simulink model "Vorlage_Prozessgut_Jaeho"  (R2022a)
settings: Solver=ode3  StartTime=0.0  StopTime=50  FixedStep=0.01  RelTol=1e-3  EnableMultiTasking=on
undefined symbols (not defined in the file): MaxFlaschen
libraries: simulink x19
settings Model: Creator=merz  LastModifiedBy=mwjae
settings SolverCC: ZeroCrossAlgorithm=Non-adaptive  AlgebraicLoopSolver=TrustRegion
settings DataIOCC: LimitDataPoints=on  SaveFormat=Array  SignalLoggingSaveFormat=ModelDataLogs  ReturnWorkspaceOutputs=off  SignalLoggingName=sigsOut
settings OptimizationCC: ExpressionDepthLimit=2147483647  InitFltsAndDblsToZero=on  LifeSpan=inf
settings DebuggingCC: SaveWithParameterizedLinksMsg=none  UnderspecifiedInitializationDetection=Classic  MergeDetectMultiDrivingBlocksExec=none  SignalResolutionControl=TryResolveAllWithWarning  MultiTaskDSMMsg=warning  MultiTaskCondExecSysMsg=none  FcnCallInpInsideContextMsg=warning  UnconnectedInputMsg=warning  UnconnectedOutputMsg=warning  UnconnectedLineMsg=warning  StateNameClashWarn=warning  SFUnexpectedBacktrackingDiag=warning  SFNoUnconditionalDefaultTransitionDiag=warning  SFExecutionAtInitializationDiag=none  SFMachineParentedDataDiag=warning  ArithmeticOperatorsInVariantConditions=warning
settings HardwareCC: ProdBitPerPointer=32  ProdBitPerSizeT=32  ProdBitPerPtrDiffT=32  ProdLargestAtomicFloat=None  ProdIntDivRoundTo=Undefined  ProdEndianess=Unspecified  ProdWordSize=32  ProdHWDeviceType=32-bit Generic  TargetUnknown=on
settings ModelReferenceCC: PropagateSignalLabelsOutOfModel=off
settings RTWCC: DLArmComputeVersion=19.05
settings CodeAppCC: StateflowObjectComments=on
settings GRTTargetCC: TargetFcnLib=ansi_tfl_tmw.mat  TargetLangStandard=C89/C90 (ANSI)  ModelReferenceCompliant=off  CombineOutputUpdateFcns=off  MatFileLogging=off  GRTInterface=on
settings ConfigComp: CovMetricSettings=dw  CovSaveCumulativeToWorkspaceVar=on  CovSaveSingleToWorkspaceVar=on

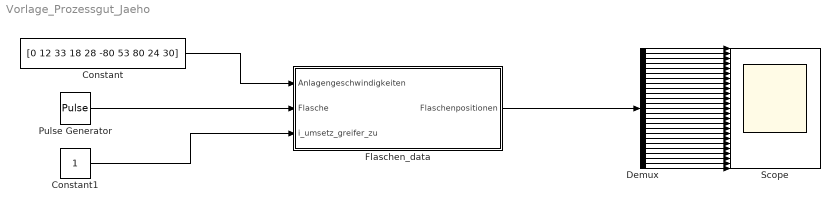
== system Vorlage_Prozessgut_Jaeho ==
  Constant : Constant  Value=[0 12 33 18 28 -80 53 80 24 30]
  Constant1 : Constant
  Demux : Demux  Outputs=25
  Flaschen_data : Subsystem
  Pulse Generator : DiscretePulseGenerator  PulseType=Time based  PulseWidth=10
  Scope : Scope  NumInputPorts=25
  wires:
  Pulse Generator/1 -> Flaschen_data/2(Flasche)
  Constant1/1 -> Flaschen_data/3(i_umsetz_greifer_zu)
  Constant/1 -> Flaschen_data/1(Anlagengeschwindigkeiten)
  Demux/2 -> Scope/2
  Demux/22 -> Scope/22
  Demux/16 -> Scope/16
  Demux/20 -> Scope/20
  Demux/5 -> Scope/5
  Demux/7 -> Scope/7
  Demux/19 -> Scope/19
  Demux/10 -> Scope/10
  Demux/9 -> Scope/9
  Demux/17 -> Scope/17
  Demux/15 -> Scope/15
  Demux/11 -> Scope/11
  Demux/8 -> Scope/8
  Demux/6 -> Scope/6
  Demux/3 -> Scope/3
  Demux/13 -> Scope/13
  Demux/25 -> Scope/25
  Demux/14 -> Scope/14
  Demux/1 -> Scope/1
  Demux/24 -> Scope/24
  Demux/4 -> Scope/4
  Demux/18 -> Scope/18
  Flaschen_data/1(Flaschenpositionen) -> Demux/1
  Demux/23 -> Scope/23
  Demux/12 -> Scope/12
  Demux/21 -> Scope/21

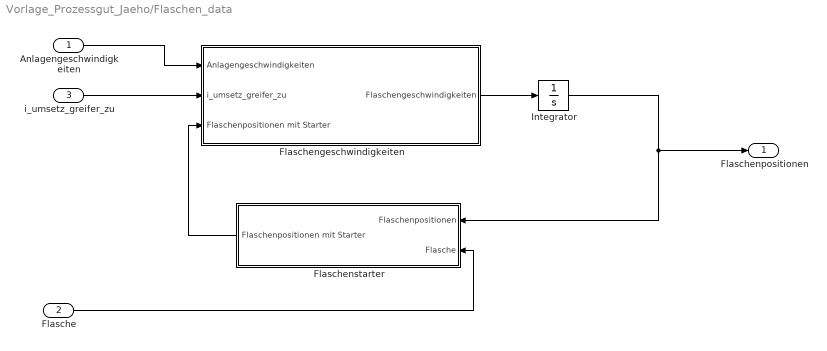
== system Vorlage_Prozessgut_Jaeho/Flaschen_data ==
  Anlagengeschwindigkeiten : Inport
  Flasche : Inport  Port=2
  i_umsetz_greifer_zu : Inport  Port=3
  Flaschengeschwindigkeiten : Subsystem
  Flaschenstarter : Subsystem
  Integrator : Integrator
  Flaschenpositionen : Outport
  wires:
  Anlagengeschwindigkeiten/1 -> Flaschengeschwindigkeiten/1(Anlagengeschwindigkeiten)
  i_umsetz_greifer_zu/1 -> Flaschengeschwindigkeiten/2(i_umsetz_greifer_zu)
  Flaschenstarter/1(Flaschenpositionen mit Starter) -> Flaschengeschwindigkeiten/3(Flaschenpositionen mit Starter)
  Flasche/1 -> Flaschenstarter/2(Flasche)
  Flaschengeschwindigkeiten/1(Flaschengeschwindigkeiten) -> Integrator/1
  Integrator/1 -> Flaschenstarter/1(Flaschenpositionen), Flaschenpositionen/1

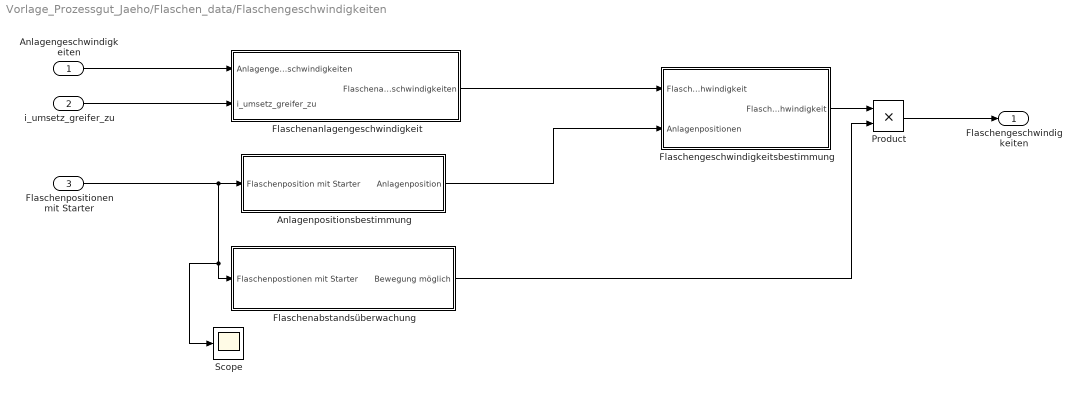
== system Vorlage_Prozessgut_Jaeho/Flaschen_data/Flaschengeschwindigkeiten ==
  Anlagengeschwindigkeiten : Inport
  i_umsetz_greifer_zu : Inport  Port=2
  Flaschenpositionen mit Starter : Inport  Port=3
  Anlagenpositionsbestimmung : Subsystem
  Flaschenabstandsüberwachung : Subsystem
  Flaschenanlagengeschwindigkeit : Subsystem
  "Flaschengeschwindigkeitsbestimmung " : Subsystem  TreatAsAtomicUnit=on
  Product : Product
  Scope : Scope
  Flaschengeschwindigkeiten : Outport
  wires:
  Anlagengeschwindigkeiten/1 -> Flaschenanlagengeschwindigkeit/1(Anlagengeschwindigkeiten)
  i_umsetz_greifer_zu/1 -> Flaschenanlagengeschwindigkeit/2(i_umsetz_greifer_zu)
  Flaschenanlagengeschwindigkeit/1(Flaschenanlagengeschwindigkeiten) -> "Flaschengeschwindigkeitsbestimmung "/1(Flaschenanlagengeschwindigkeit)
  Anlagenpositionsbestimmung/1(Anlagenposition) -> "Flaschengeschwindigkeitsbestimmung "/2(Anlagenpositionen)
  Flaschenpositionen mit Starter/1 -> Scope/1, Flaschenabstandsüberwachung/1(Flaschenpostionen mit Starter), Anlagenpositionsbestimmung/1(Flaschenposition mit Starter)
  "Flaschengeschwindigkeitsbestimmung "/1(Flaschengeschwindigkeit) -> Product/1
  Flaschenabstandsüberwachung/1(Bewegung möglich) -> Product/2
  Product/1 -> Flaschengeschwindigkeiten/1

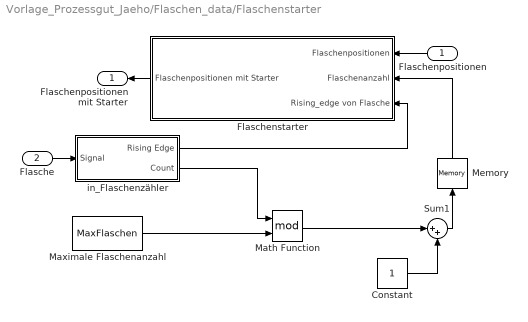
== system Vorlage_Prozessgut_Jaeho/Flaschen_data/Flaschenstarter ==
  Flaschenpositionen : Inport
  Flasche : Inport  Port=2
  Constant : Constant  OutDataTypeStr=uint16
  Flaschenstarter : Subsystem
  Math Function : Math  Operator=mod  SignedPower=on
  Maximale Flaschenanzahl : Constant  Value=MaxFlaschen  OutDataTypeStr=uint16
  Memory : Memory  InitialCondition=1
  Sum1 : Sum  Inputs=|++  SaturateOnIntegerOverflow=on
  in_Flaschenzähler : Subsystem
  Flaschenpositionen mit Starter : Outport
  wires:
  in_Flaschenzähler/2(Count) -> Math Function/1
  Maximale Flaschenanzahl/1 -> Math Function/2
  Math Function/1 -> Sum1/1
  in_Flaschenzähler/1(Rising Edge) -> Flaschenstarter/3(Rising_edge von Flasche)
  Sum1/1 -> Memory/1
  Constant/1 -> Sum1/2
  Memory/1 -> Flaschenstarter/2(Flaschenanzahl)
  Flaschenpositionen/1 -> Flaschenstarter/1(Flaschenpositionen)
  Flaschenstarter/1(Flaschenpositionen mit Starter) -> Flaschenpositionen mit Starter/1
  Flasche/1 -> in_Flaschenzähler/1(Signal)

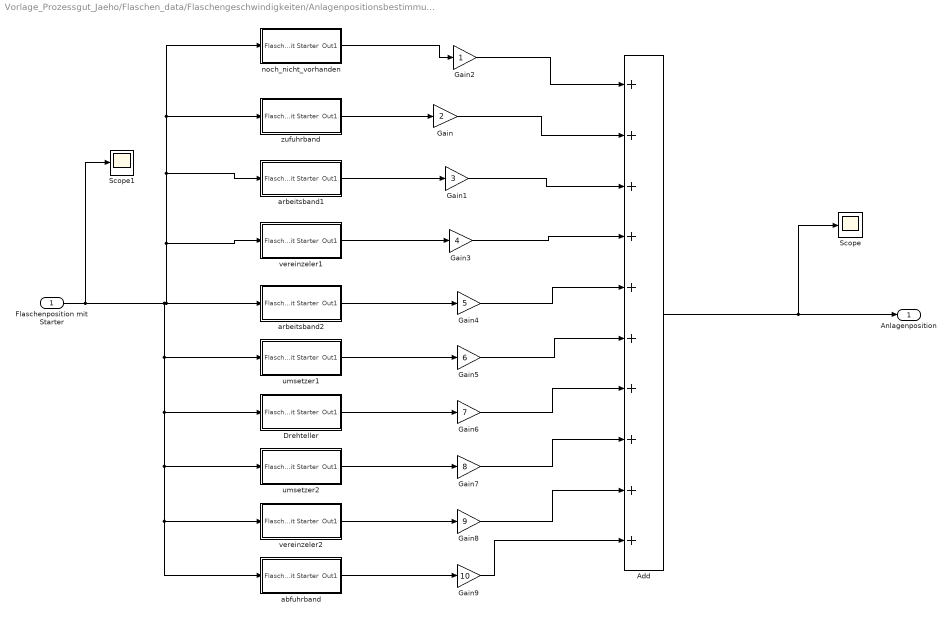
== system Vorlage_Prozessgut_Jaeho/Flaschen_data/Flaschengeschwindigkeiten/Anlagenpositionsbestimmung ==
  Flaschenposition mit Starter : Inport
  Add : Sum  Inputs=++++++++++
  Drehteller : Subsystem
  Gain : Gain  Gain=2
  Gain1 : Gain  Gain=3
  Gain2 : Gain
  Gain3 : Gain  Gain=4
  Gain4 : Gain  Gain=5
  Gain5 : Gain  Gain=6
  Gain6 : Gain  Gain=7
  Gain7 : Gain  Gain=8
  Gain8 : Gain  Gain=9
  Gain9 : Gain  Gain=10
  Scope : Scope
  Scope1 : Scope
  abfuhrband : Subsystem
  arbeitsband1 : Subsystem
  arbeitsband2 : Subsystem
  noch_nicht_vorhanden : Subsystem
  umsetzer1 : Subsystem
  umsetzer2 : Subsystem
  vereinzeler1 : Subsystem
  vereinzeler2 : Subsystem
  zufuhrband : Subsystem
  Anlagenposition : Outport
  wires:
  Flaschenposition mit Starter/1 -> Scope1/1, abfuhrband/1(Flaschenposition mit Starter), vereinzeler2/1(Flaschenposition mit Starter), umsetzer2/1(Flaschenposition mit Starter), Drehteller/1(Flaschenposition mit Starter), umsetzer1/1(Flaschenposition mit Starter), vereinzeler1/1(Flaschenposition mit Starter), arbeitsband1/1(Flaschenposition mit Starter), zufuhrband/1(Flaschenposition mit Starter), noch_nicht_vorhanden/1(Flaschenposition mit Starter), arbeitsband2/1(Flaschenposition mit Starter)
  Add/1 -> Scope/1, Anlagenposition/1
  Gain/1 -> Add/2
  Gain1/1 -> Add/3
  Gain2/1 -> Add/1
  Gain3/1 -> Add/4
  Gain4/1 -> Add/5
  Gain5/1 -> Add/6
  Gain6/1 -> Add/7
  Gain7/1 -> Add/8
  Gain8/1 -> Add/9
  Gain9/1 -> Add/10
  noch_nicht_vorhanden/1(Out1) -> Gain2/1
  zufuhrband/1(Out1) -> Gain/1
  arbeitsband1/1(Out1) -> Gain1/1
  vereinzeler1/1(Out1) -> Gain3/1
  arbeitsband2/1(Out1) -> Gain4/1
  umsetzer1/1(Out1) -> Gain5/1
  Drehteller/1(Out1) -> Gain6/1
  umsetzer2/1(Out1) -> Gain7/1
  vereinzeler2/1(Out1) -> Gain8/1
  abfuhrband/1(Out1) -> Gain9/1

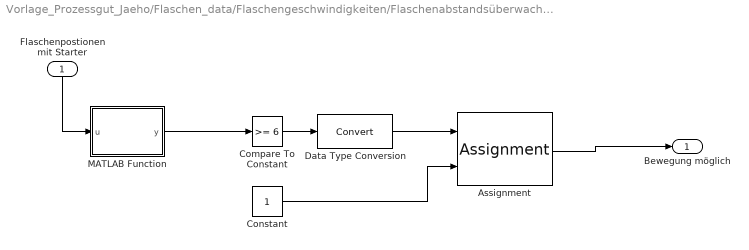
== system Vorlage_Prozessgut_Jaeho/Flaschen_data/Flaschengeschwindigkeiten/Flaschenabstandsüberwachung ==
  Flaschenpostionen mit Starter : Inport
  Assignment : Assignment  DiagnosticForDimensions=Warning  IndexOptions=Index vector (dialog)  Indices=1  OutputSizes=1
  Compare To Constant : simulink/Logic and Bit Operations/Compare To Constant  relop=>=  const=6  OutDataTypeStr=boolean
  Constant : Constant
  Data Type Conversion : DataTypeConversion  SaturateOnIntegerOverflow=off  RndMeth=Floor
  MATLAB Function : MATLAB Function  TreatAsAtomicUnit=on
  Bewegung möglich : Outport
  wires:
  Flaschenpostionen mit Starter/1 -> MATLAB Function/1(u)
  MATLAB Function/1(y) -> Compare To Constant/1
  Compare To Constant/1 -> Data Type Conversion/1
  Constant/1 -> Assignment/2
  Assignment/1 -> Bewegung möglich/1
  Data Type Conversion/1 -> Assignment/1

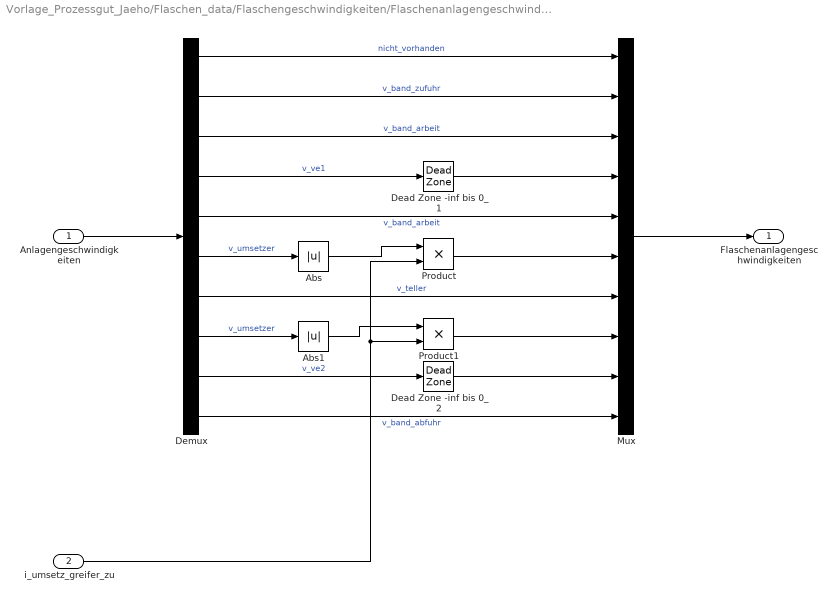
== system Vorlage_Prozessgut_Jaeho/Flaschen_data/Flaschengeschwindigkeiten/Flaschenanlagengeschwindigkeit ==
  Anlagengeschwindigkeiten : Inport
  i_umsetz_greifer_zu : Inport  Port=2
  Abs : Abs  SaturateOnIntegerOverflow=off
  Abs1 : Abs  SaturateOnIntegerOverflow=off
  Dead Zone -inf bis 0_1 : DeadZone  LowerValue=-inf  UpperValue=0
  Dead Zone -inf bis 0_2 : DeadZone  LowerValue=-inf  UpperValue=0
  Demux : Demux  Outputs=10
  Mux : Mux  Inputs=10
  Product : Product
  Product1 : Product
  Flaschenanlagengeschwindigkeiten : Outport
  wires:
  Anlagengeschwindigkeiten/1 -> Demux/1
  Demux/1 -> Mux/1  "nicht_vorhanden"
  Demux/2 -> Mux/2  "v_band_zufuhr"
  Demux/3 -> Mux/3  "v_band_arbeit"
  Demux/4 -> Dead Zone -inf bis 0_1/1  "v_ve1"
  Demux/5 -> Mux/5  "v_band_arbeit"
  Demux/6 -> Abs/1  "v_umsetzer"
  Demux/7 -> Mux/7  "v_teller"
  Demux/8 -> Abs1/1  "v_umsetzer"
  Demux/10 -> Mux/10  "v_band_abfuhr"
  Dead Zone -inf bis 0_1/1 -> Mux/4
  Dead Zone -inf bis 0_2/1 -> Mux/9
  Demux/9 -> Dead Zone -inf bis 0_2/1  "v_ve2"
  Abs/1 -> Product/1
  i_umsetz_greifer_zu/1 -> Product1/2, Product/2
  Abs1/1 -> Product1/1
  Product/1 -> Mux/6
  Product1/1 -> Mux/8
  Mux/1 -> Flaschenanlagengeschwindigkeiten/1

== system Vorlage_Prozessgut_Jaeho/Flaschen_data/Flaschengeschwindigkeiten/Flaschengeschwindigkeitsbestimmung  ==
  Flaschenanlagengeschwindigkeit : Inport
  Anlagenpositionen : Inport  Port=2
  Selector : Selector  InputPortWidth=10  IndexOptions=Index vector (port)  Indices=[1 3]  OutputSizes=1
  Flaschengeschwindigkeit : Outport
  wires:
  Flaschenanlagengeschwindigkeit/1 -> Selector/1
  Anlagenpositionen/1 -> Selector/2
  Selector/1 -> Flaschengeschwindigkeit/1

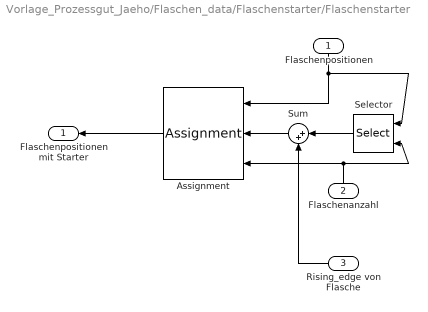
== system Vorlage_Prozessgut_Jaeho/Flaschen_data/Flaschenstarter/Flaschenstarter ==
  Flaschenpositionen : Inport
  Flaschenanzahl : Inport  Port=2
  Rising_edge von Flasche : Inport  Port=3
  Assignment : Assignment  IndexOptions=Index vector (port)  Indices=1  OutputSizes=[1]
  Selector : Selector  InputPortWidth=MaxFlaschen  IndexOptions=Index vector (port)  Indices=[1 3]  OutputSizes=1
  Sum : Sum  Inputs=|++  OutDataTypeStr=double  RndMeth=Zero
  Flaschenpositionen mit Starter : Outport
  wires:
  Selector/1 -> Sum/1
  Sum/1 -> Assignment/2
  Flaschenanzahl/1 -> Selector/2, Assignment/3
  Flaschenpositionen/1 -> Assignment/1, Selector/1
  Assignment/1 -> Flaschenpositionen mit Starter/1
  Rising_edge von Flasche/1 -> Sum/2

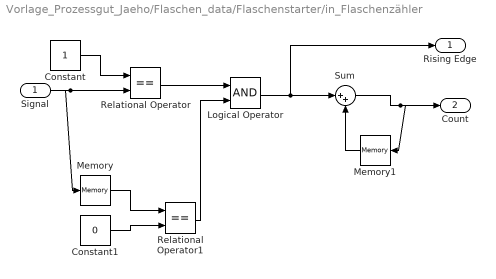
== system Vorlage_Prozessgut_Jaeho/Flaschen_data/Flaschenstarter/in_Flaschenzähler ==
  Signal : Inport
  Constant : Constant
  Constant1 : Constant  Value=0
  Logical Operator : Logic  AllPortsSameDT=off
  Memory : Memory
  Memory1 : Memory
  Relational Operator : RelationalOperator  Operator===  InputSameDT=off
  Relational Operator1 : RelationalOperator  Operator===  InputSameDT=off
  Sum : Sum  Inputs=|++  OutDataTypeStr=uint16  SaturateOnIntegerOverflow=on
  Rising Edge : Outport
  Count : Outport  Port=2
  wires:
  Signal/1 -> Memory/1, Relational Operator/2
  Constant/1 -> Relational Operator/1
  Relational Operator/1 -> Logical Operator/1
  Constant1/1 -> Relational Operator1/2
  Memory/1 -> Relational Operator1/1
  Relational Operator1/1 -> Logical Operator/2
  Logical Operator/1 -> Sum/1, Rising Edge/1
  Memory1/1 -> Sum/2
  Sum/1 -> Count/1, Memory1/1

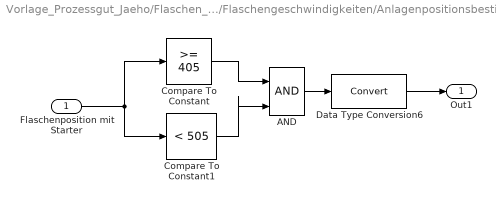
== system Vorlage_Prozessgut_Jaeho/Flaschen_data/Flaschengeschwindigkeiten/Anlagenpositionsbestimmung/Drehteller ==
  Flaschenposition mit Starter : Inport
  AND : Logic  IconShape=distinctive  AllPortsSameDT=off  OutDataTypeStr=boolean
  Compare To Constant : simulink/Logic and Bit Operations/Compare To Constant  relop=>=  const=405  OutDataTypeStr=boolean
  Compare To Constant1 : simulink/Logic and Bit Operations/Compare To Constant  relop=<  const=505  OutDataTypeStr=boolean
  Data Type Conversion6 : DataTypeConversion  SaturateOnIntegerOverflow=off  RndMeth=Floor
  Out1 : Outport
  wires:
  Flaschenposition mit Starter/1 -> Compare To Constant1/1, Compare To Constant/1
  Compare To Constant/1 -> AND/1
  Compare To Constant1/1 -> AND/2
  AND/1 -> Data Type Conversion6/1
  Data Type Conversion6/1 -> Out1/1

== system Vorlage_Prozessgut_Jaeho/Flaschen_data/Flaschengeschwindigkeiten/Anlagenpositionsbestimmung/abfuhrband ==
  Flaschenposition mit Starter : Inport
  Compare To Constant : simulink/Logic and Bit Operations/Compare To Constant  relop=>=  const=610  OutDataTypeStr=boolean
  Data Type Conversion9 : DataTypeConversion  SaturateOnIntegerOverflow=off  RndMeth=Floor
  Out1 : Outport
  wires:
  Flaschenposition mit Starter/1 -> Compare To Constant/1
  Compare To Constant/1 -> Data Type Conversion9/1
  Data Type Conversion9/1 -> Out1/1

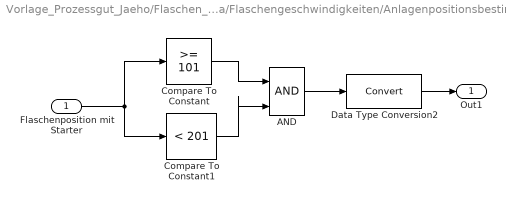
== system Vorlage_Prozessgut_Jaeho/Flaschen_data/Flaschengeschwindigkeiten/Anlagenpositionsbestimmung/arbeitsband1 ==
  Flaschenposition mit Starter : Inport
  AND : Logic  IconShape=distinctive  AllPortsSameDT=off  OutDataTypeStr=boolean
  Compare To Constant : simulink/Logic and Bit Operations/Compare To Constant  relop=>=  const=101  OutDataTypeStr=boolean
  Compare To Constant1 : simulink/Logic and Bit Operations/Compare To Constant  relop=<  const=201  OutDataTypeStr=boolean
  Data Type Conversion2 : DataTypeConversion  SaturateOnIntegerOverflow=off  RndMeth=Floor
  Out1 : Outport
  wires:
  Flaschenposition mit Starter/1 -> Compare To Constant1/1, Compare To Constant/1
  Compare To Constant/1 -> AND/1
  Compare To Constant1/1 -> AND/2
  AND/1 -> Data Type Conversion2/1
  Data Type Conversion2/1 -> Out1/1

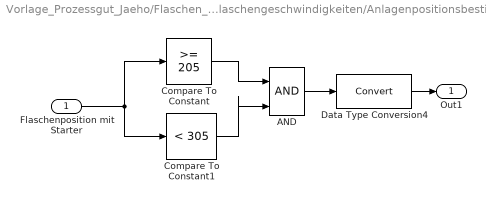
== system Vorlage_Prozessgut_Jaeho/Flaschen_data/Flaschengeschwindigkeiten/Anlagenpositionsbestimmung/arbeitsband2 ==
  Flaschenposition mit Starter : Inport
  AND : Logic  IconShape=distinctive  AllPortsSameDT=off  OutDataTypeStr=boolean
  Compare To Constant : simulink/Logic and Bit Operations/Compare To Constant  relop=>=  const=205  OutDataTypeStr=boolean
  Compare To Constant1 : simulink/Logic and Bit Operations/Compare To Constant  relop=<  const=305  OutDataTypeStr=boolean
  Data Type Conversion4 : DataTypeConversion  SaturateOnIntegerOverflow=off  RndMeth=Floor
  Out1 : Outport
  wires:
  Flaschenposition mit Starter/1 -> Compare To Constant1/1, Compare To Constant/1
  Compare To Constant/1 -> AND/1
  Compare To Constant1/1 -> AND/2
  AND/1 -> Data Type Conversion4/1
  Data Type Conversion4/1 -> Out1/1

== system Vorlage_Prozessgut_Jaeho/Flaschen_data/Flaschengeschwindigkeiten/Anlagenpositionsbestimmung/noch_nicht_vorhanden ==
  Flaschenposition mit Starter : Inport
  Compare To Constant : simulink/Logic and Bit Operations/Compare To Constant  relop=<=  const=0  OutDataTypeStr=boolean
  Data Type Conversion3 : DataTypeConversion  SaturateOnIntegerOverflow=off  RndMeth=Floor
  Out1 : Outport
  wires:
  Flaschenposition mit Starter/1 -> Compare To Constant/1
  Compare To Constant/1 -> Data Type Conversion3/1
  Data Type Conversion3/1 -> Out1/1

== system Vorlage_Prozessgut_Jaeho/Flaschen_data/Flaschengeschwindigkeiten/Anlagenpositionsbestimmung/umsetzer1 ==
  Flaschenposition mit Starter : Inport
  AND : Logic  IconShape=distinctive  AllPortsSameDT=off  OutDataTypeStr=boolean
  Compare To Constant : simulink/Logic and Bit Operations/Compare To Constant  relop=>=  const=305  OutDataTypeStr=boolean
  Compare To Constant1 : simulink/Logic and Bit Operations/Compare To Constant  relop=<  const=405  OutDataTypeStr=boolean
  Data Type Conversion5 : DataTypeConversion  SaturateOnIntegerOverflow=off  RndMeth=Floor
  Out1 : Outport
  wires:
  Flaschenposition mit Starter/1 -> Compare To Constant1/1, Compare To Constant/1
  Compare To Constant/1 -> AND/1
  Compare To Constant1/1 -> AND/2
  AND/1 -> Data Type Conversion5/1
  Data Type Conversion5/1 -> Out1/1

== system Vorlage_Prozessgut_Jaeho/Flaschen_data/Flaschengeschwindigkeiten/Anlagenpositionsbestimmung/umsetzer2 ==
  Flaschenposition mit Starter : Inport
  AND : Logic  IconShape=distinctive  AllPortsSameDT=off  OutDataTypeStr=boolean
  Compare To Constant : simulink/Logic and Bit Operations/Compare To Constant  relop=>=  const=505  OutDataTypeStr=boolean
  Compare To Constant1 : simulink/Logic and Bit Operations/Compare To Constant  relop=<  const=605  OutDataTypeStr=boolean
  Data Type Conversion7 : DataTypeConversion  SaturateOnIntegerOverflow=off  RndMeth=Floor
  Out1 : Outport
  wires:
  Flaschenposition mit Starter/1 -> Compare To Constant1/1, Compare To Constant/1
  Compare To Constant/1 -> AND/1
  Compare To Constant1/1 -> AND/2
  AND/1 -> Data Type Conversion7/1
  Data Type Conversion7/1 -> Out1/1

== system Vorlage_Prozessgut_Jaeho/Flaschen_data/Flaschengeschwindigkeiten/Anlagenpositionsbestimmung/vereinzeler1 ==
  Flaschenposition mit Starter : Inport
  AND : Logic  IconShape=distinctive  AllPortsSameDT=off  OutDataTypeStr=boolean
  Compare To Constant : simulink/Logic and Bit Operations/Compare To Constant  relop=>=  const=201  OutDataTypeStr=boolean
  Compare To Constant1 : simulink/Logic and Bit Operations/Compare To Constant  relop=<  const=205  OutDataTypeStr=boolean
  Data Type Conversion3 : DataTypeConversion  SaturateOnIntegerOverflow=off  RndMeth=Floor
  Out1 : Outport
  wires:
  Flaschenposition mit Starter/1 -> Compare To Constant1/1, Compare To Constant/1
  Compare To Constant/1 -> AND/1
  Compare To Constant1/1 -> AND/2
  AND/1 -> Data Type Conversion3/1
  Data Type Conversion3/1 -> Out1/1

== system Vorlage_Prozessgut_Jaeho/Flaschen_data/Flaschengeschwindigkeiten/Anlagenpositionsbestimmung/vereinzeler2 ==
  Flaschenposition mit Starter : Inport
  AND : Logic  IconShape=distinctive  AllPortsSameDT=off  OutDataTypeStr=boolean
  Compare To Constant : simulink/Logic and Bit Operations/Compare To Constant  relop=>=  const=605  OutDataTypeStr=boolean
  Compare To Constant1 : simulink/Logic and Bit Operations/Compare To Constant  relop=<  const=610  OutDataTypeStr=boolean
  Data Type Conversion8 : DataTypeConversion  SaturateOnIntegerOverflow=off  RndMeth=Floor
  Out1 : Outport
  wires:
  Flaschenposition mit Starter/1 -> Compare To Constant1/1, Compare To Constant/1
  Compare To Constant/1 -> AND/1
  Compare To Constant1/1 -> AND/2
  AND/1 -> Data Type Conversion8/1
  Data Type Conversion8/1 -> Out1/1

== system Vorlage_Prozessgut_Jaeho/Flaschen_data/Flaschengeschwindigkeiten/Anlagenpositionsbestimmung/zufuhrband ==
  Flaschenposition mit Starter : Inport
  AND : Logic  IconShape=distinctive  AllPortsSameDT=off  OutDataTypeStr=boolean
  Compare To Constant : simulink/Logic and Bit Operations/Compare To Constant  relop=>  const=0  OutDataTypeStr=boolean
  Compare To Constant1 : simulink/Logic and Bit Operations/Compare To Constant  relop=<  const=101  OutDataTypeStr=boolean
  Data Type Conversion1 : DataTypeConversion  SaturateOnIntegerOverflow=off  RndMeth=Floor
  Out1 : Outport
  wires:
  Flaschenposition mit Starter/1 -> Compare To Constant1/1, Compare To Constant/1
  Compare To Constant/1 -> AND/1
  Compare To Constant1/1 -> AND/2
  AND/1 -> Data Type Conversion1/1
  Data Type Conversion1/1 -> Out1/1

== matlab function Vorlage_Prozessgut_Jaeho/Flaschen_data/Flaschengeschwindigkeiten/Flaschenabstandsüberwachung/MATLAB Function ==
  data: u input; y output
function y = fcn(u)

y = circshift(u,1)-u;
